simulink model "quadcopter_model"  (R2023a)
settings: Solver=odeN  StartTime=0.0  StopTime=20  MaxStep=0.2  RelTol=1e-3
libraries: slpidlib x3
settings Model: Creator=Lenovo  LastModifiedBy=Lenovo
settings SolverCC: MaxConsecutiveMinStep=5

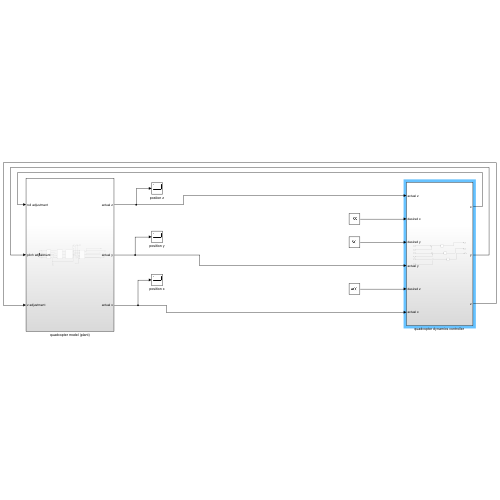
[thumbnail: Simulink's stored preview of the top-level diagram]
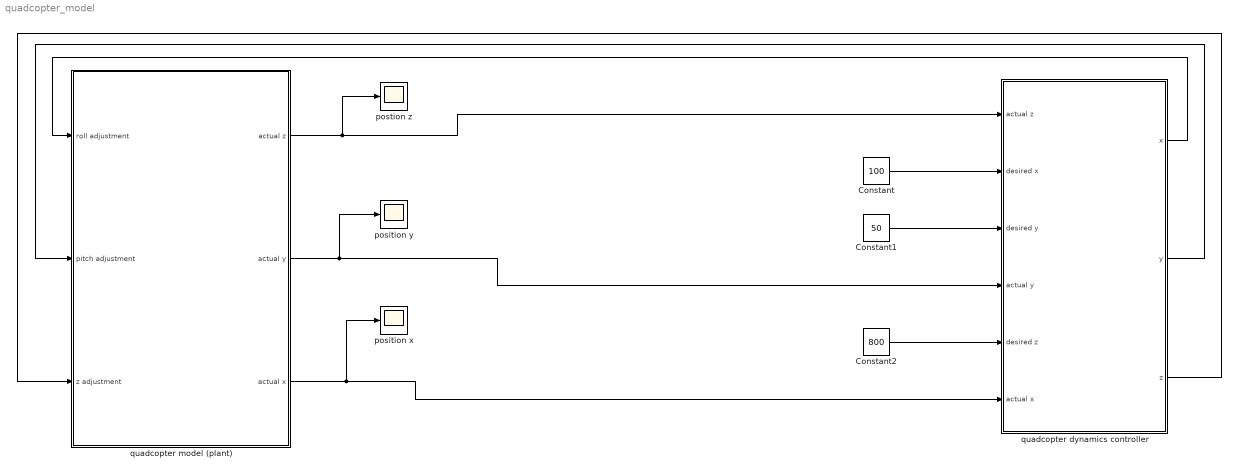
== system quadcopter_model ==
  Constant : Constant  Value=100
  Constant1 : Constant  Value=50
  Constant2 : Constant  Value=800
  position x : Scope
  position y : Scope
  postion z : Scope
  "quadcopter dynamics controller " : Subsystem
  quadcopter model (plant) : Subsystem
  wires:
  "quadcopter dynamics controller "/3(z) -> quadcopter model (plant)/3(z adjustment)
  "quadcopter dynamics controller "/2(y) -> quadcopter model (plant)/2("pitch adjustment ")
  "quadcopter dynamics controller "/1(x) -> quadcopter model (plant)/1(roll adjustment)
  quadcopter model (plant)/1(actual z) -> postion z/1, "quadcopter dynamics controller "/1(actual z)
  quadcopter model (plant)/2(actual y) -> position y/1, "quadcopter dynamics controller "/4(actual y)
  quadcopter model (plant)/3(actual x) -> position x/1, "quadcopter dynamics controller "/6(actual x)
  Constant1/1 -> "quadcopter dynamics controller "/3(desired y)
  Constant/1 -> "quadcopter dynamics controller "/2(desired x)
  Constant2/1 -> "quadcopter dynamics controller "/5(desired z)

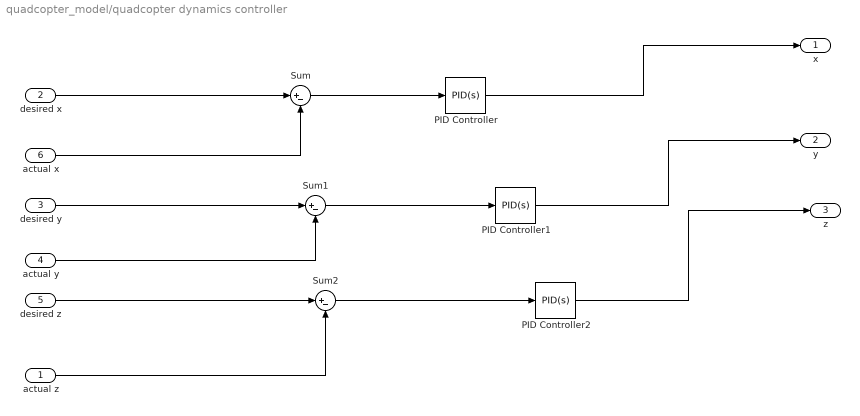
== system quadcopter_model/quadcopter dynamics controller  ==
  actual z : Inport
  desired x : Inport  Port=2
  desired y : Inport  Port=3
  actual y : Inport  Port=4
  desired z : Inport  Port=5
  actual x : Inport  Port=6
  PID Controller : slpidlib/PID Controller  Controller=PID  Form=Parallel  TimeDomain=Continuous-time  UseExternalTs=off  SampleTime=-1  IntegratorMethod=Forward Euler  FilterMethod=Forward Euler  ControllerParametersSource=internal  P=5.80247697722311e-07  I=2.71641673162191e-08  UseKiTs=on  D=3.04350306749436e-06  N=5.45397025421619  UseFilter=on  TunerSelectOption=Transfer Function Based (PID Tuner App)  InitialConditionSource=internal  InitialConditionForIntegrator=0  InitialConditionForFilter=0  DifferentiatorICPrevScaledInput=0  ExternalReset=none  TrackingMode=off  Kt=1  LimitOutput=off  SatLimitsSource=internal  UpperSaturationLimit=inf  LowerSaturationLimit=-inf  LinearizeAsGain=on  AntiWindupMode=none  Kb=1  LimitIntegrator=off  UpperIntegratorSaturationLimit=inf  LowerIntegratorSaturationLimit=-inf  POutMin=[]  POutMax=[]  IOutMin=[]  IOutMax=[]  DOutMin=[]  DOutMax=[]  NOutMin=[]  NOutMax=[]  SumOutMin=[]  SumOutMax=[]  SaturationOutMin=[]  SaturationOutMax=[]  PParamMin=[]  PParamMax=[]  IParamMin=[]  IParamMax=[]  DParamMin=[]  DParamMax=[]  NParamMin=[]  NParamMax=[]  KbParamMin=[]  KbParamMax=[]  KtParamMin=[]  KtParamMax=[]  KbOutMin=[]  KbOutMax=[]  KtOutMin=[]  KtOutMax=[]  IntegratorOutMin=[]  IntegratorOutMax=[]  FilterOutMin=[]  FilterOutMax=[]  SumI1OutMin=[]  SumI1OutMax=[]  SumI2OutMin=[]  SumI2OutMax=[]  SumI3OutMin=[]  SumI3OutMax=[]  SumI4OutMin=[]  SumI4OutMax=[]  SumDOutMin=[]  SumDOutMax=[]  DifferentiatorOutMin=[]  DifferentiatorOutMax=[]  FilterDiffOutCoefMin=[]  FilterDiffOutCoefMax=[]  ReciprocalOutMin=[]  ReciprocalOutMax=[]  SumDenOutMin=[]  SumDenOutMax=[]  SumNumOutMin=[]  SumNumOutMax=[]  DivideOutMin=[]  DivideOutMax=[]  UdiffTsProdOutMin=[]  UdiffTsProdOutMax=[]  NTsProdOutMin=[]  NTsProdOutMax=[]  UintegralTsProdOutMin=[]  UintegralTsProdOutMax=[]  UngainTsProdOutMin=[]  UngainTsProdOutMax=[]  ClampingZeroOutDataTypeStr=Inherit: Inherit via back propagation  ClampingZeroOutMin=[]  ClampingZeroOutMax=[]  FilterDenConstantOutDataTypeStr=Inherit: Inherit via back propagation  FilterDenConstantOutMin=[]  FilterDenConstantOutMax=[]  PCopyOutDataTypeStr=Inherit: Inherit via back propagation  PCopyOutMin=[]  PCopyOutMax=[]  NCopyOutDataTypeStr=Inherit: Inherit via back propagation  NCopyOutMin=[]  NCopyOutMax=[]  IntegratorContinuousStateAttributes=''  IntegratorStateMustResolveToSignalObject=off  IntegratorRTWStateStorageClass=Auto  FilterContinuousStateAttributes=''  FilterStateMustResolveToSignalObject=off  FilterRTWStateStorageClass=Auto  ParallelPVariant=InternalParameters  IdealPVariant=Disabled  IVariant=InternalParameters  DVariant=InternalParameters  IntegratorVariant=Continuous  SatVariant=Disabled  AWVariant=Passthrough  PCopyVariant=Disabled  TRVariant=Disabled  FdbkBlocksVariant=Forward  IdealPFdbkVariant=Disabled  SatFdbkVariant=Disabled  DerivativeFilterVariant=ContFilter  NVariant=InternalParameters  NCopyVariant=Disabled  FilterICVariant=InternalICsFilter  IntegratorICVariant=InternalICs  ExternalResetVariant=Disabled  TRSumVariant=Passthrough  SumFdbkVariant=Disabled  SumVariant=Sum_PID  TsampFilterVariant=InternalTs  TsampNgainVariant=Passthrough  TsampIntegralVariant=Disabled_SignalSpec  ExternalSaturationOutDataTypeStr=Inherit: Same as second input
  PID Controller1 : slpidlib/PID Controller  Controller=PID  Form=Ideal  TimeDomain=Continuous-time  UseExternalTs=off  SampleTime=-1  IntegratorMethod=Forward Euler  FilterMethod=Forward Euler  ControllerParametersSource=internal  P=-5.80247697722311e-07  I=0.0468147782797737  UseKiTs=on  D=5.24517904929436  N=5.45397025421619  UseFilter=on  TunerSelectOption=Transfer Function Based (PID Tuner App)  InitialConditionSource=internal  InitialConditionForIntegrator=0  InitialConditionForFilter=0  DifferentiatorICPrevScaledInput=0  ExternalReset=none  TrackingMode=off  Kt=1  LimitOutput=off  SatLimitsSource=internal  UpperSaturationLimit=inf  LowerSaturationLimit=-inf  LinearizeAsGain=on  AntiWindupMode=none  Kb=1  LimitIntegrator=off  UpperIntegratorSaturationLimit=inf  LowerIntegratorSaturationLimit=-inf  POutMin=[]  POutMax=[]  IOutMin=[]  IOutMax=[]  DOutMin=[]  DOutMax=[]  NOutMin=[]  NOutMax=[]  SumOutMin=[]  SumOutMax=[]  SaturationOutMin=[]  SaturationOutMax=[]  PParamMin=[]  PParamMax=[]  IParamMin=[]  IParamMax=[]  DParamMin=[]  DParamMax=[]  NParamMin=[]  NParamMax=[]  KbParamMin=[]  KbParamMax=[]  KtParamMin=[]  KtParamMax=[]  KbOutMin=[]  KbOutMax=[]  KtOutMin=[]  KtOutMax=[]  IntegratorOutMin=[]  IntegratorOutMax=[]  FilterOutMin=[]  FilterOutMax=[]  SumI1OutMin=[]  SumI1OutMax=[]  SumI2OutMin=[]  SumI2OutMax=[]  SumI3OutMin=[]  SumI3OutMax=[]  SumI4OutMin=[]  SumI4OutMax=[]  SumDOutMin=[]  SumDOutMax=[]  DifferentiatorOutMin=[]  DifferentiatorOutMax=[]  FilterDiffOutCoefMin=[]  FilterDiffOutCoefMax=[]  ReciprocalOutMin=[]  ReciprocalOutMax=[]  SumDenOutMin=[]  SumDenOutMax=[]  SumNumOutMin=[]  SumNumOutMax=[]  DivideOutMin=[]  DivideOutMax=[]  UdiffTsProdOutMin=[]  UdiffTsProdOutMax=[]  NTsProdOutMin=[]  NTsProdOutMax=[]  UintegralTsProdOutMin=[]  UintegralTsProdOutMax=[]  UngainTsProdOutMin=[]  UngainTsProdOutMax=[]  ClampingZeroOutDataTypeStr=Inherit: Inherit via back propagation  ClampingZeroOutMin=[]  ClampingZeroOutMax=[]  FilterDenConstantOutDataTypeStr=Inherit: Inherit via back propagation  FilterDenConstantOutMin=[]  FilterDenConstantOutMax=[]  PCopyOutDataTypeStr=Inherit: Inherit via back propagation  PCopyOutMin=[]  PCopyOutMax=[]  NCopyOutDataTypeStr=Inherit: Inherit via back propagation  NCopyOutMin=[]  NCopyOutMax=[]  IntegratorContinuousStateAttributes=''  IntegratorStateMustResolveToSignalObject=off  IntegratorRTWStateStorageClass=Auto  FilterContinuousStateAttributes=''  FilterStateMustResolveToSignalObject=off  FilterRTWStateStorageClass=Auto  ParallelPVariant=Passthrough  IdealPVariant=InternalParameters  IVariant=InternalParameters  DVariant=InternalParameters  IntegratorVariant=Continuous  SatVariant=Disabled  AWVariant=Passthrough  PCopyVariant=Disabled  TRVariant=Disabled  FdbkBlocksVariant=Forward  IdealPFdbkVariant=Disabled  SatFdbkVariant=Disabled  DerivativeFilterVariant=ContFilter  NVariant=InternalParameters  NCopyVariant=Disabled  FilterICVariant=InternalICsFilter  IntegratorICVariant=InternalICs  ExternalResetVariant=Disabled  TRSumVariant=Passthrough  SumFdbkVariant=Disabled  SumVariant=Sum_PID  TsampFilterVariant=InternalTs  TsampNgainVariant=Passthrough  TsampIntegralVariant=Disabled_SignalSpec  ExternalSaturationOutDataTypeStr=Inherit: Same as second input
  PID Controller2 : slpidlib/PID Controller  Controller=PID  Form=Parallel  TimeDomain=Continuous-time  UseExternalTs=off  SampleTime=-1  IntegratorMethod=Forward Euler  FilterMethod=Forward Euler  ControllerParametersSource=internal  P=5.80247697722311e-07  I=2.71641673162191e-08  UseKiTs=off  D=3.04350306749436e-06  N=5.45397025421619  UseFilter=on  TunerSelectOption=Transfer Function Based (PID Tuner App)  InitialConditionSource=internal  InitialConditionForIntegrator=0  InitialConditionForFilter=0  DifferentiatorICPrevScaledInput=0  ExternalReset=none  TrackingMode=off  Kt=1  LimitOutput=off  SatLimitsSource=internal  UpperSaturationLimit=inf  LowerSaturationLimit=-inf  LinearizeAsGain=on  AntiWindupMode=none  Kb=1  LimitIntegrator=off  UpperIntegratorSaturationLimit=inf  LowerIntegratorSaturationLimit=-inf  POutMin=[]  POutMax=[]  IOutMin=[]  IOutMax=[]  DOutMin=[]  DOutMax=[]  NOutMin=[]  NOutMax=[]  SumOutMin=[]  SumOutMax=[]  SaturationOutMin=[]  SaturationOutMax=[]  PParamMin=[]  PParamMax=[]  IParamMin=[]  IParamMax=[]  DParamMin=[]  DParamMax=[]  NParamMin=[]  NParamMax=[]  KbParamMin=[]  KbParamMax=[]  KtParamMin=[]  KtParamMax=[]  KbOutMin=[]  KbOutMax=[]  KtOutMin=[]  KtOutMax=[]  IntegratorOutMin=[]  IntegratorOutMax=[]  FilterOutMin=[]  FilterOutMax=[]  SumI1OutMin=[]  SumI1OutMax=[]  SumI2OutMin=[]  SumI2OutMax=[]  SumI3OutMin=[]  SumI3OutMax=[]  SumI4OutMin=[]  SumI4OutMax=[]  SumDOutMin=[]  SumDOutMax=[]  DifferentiatorOutMin=[]  DifferentiatorOutMax=[]  FilterDiffOutCoefMin=[]  FilterDiffOutCoefMax=[]  ReciprocalOutMin=[]  ReciprocalOutMax=[]  SumDenOutMin=[]  SumDenOutMax=[]  SumNumOutMin=[]  SumNumOutMax=[]  DivideOutMin=[]  DivideOutMax=[]  UdiffTsProdOutMin=[]  UdiffTsProdOutMax=[]  NTsProdOutMin=[]  NTsProdOutMax=[]  UintegralTsProdOutMin=[]  UintegralTsProdOutMax=[]  UngainTsProdOutMin=[]  UngainTsProdOutMax=[]  ClampingZeroOutDataTypeStr=Inherit: Inherit via back propagation  ClampingZeroOutMin=[]  ClampingZeroOutMax=[]  FilterDenConstantOutDataTypeStr=Inherit: Inherit via back propagation  FilterDenConstantOutMin=[]  FilterDenConstantOutMax=[]  PCopyOutDataTypeStr=Inherit: Inherit via back propagation  PCopyOutMin=[]  PCopyOutMax=[]  NCopyOutDataTypeStr=Inherit: Inherit via back propagation  NCopyOutMin=[]  NCopyOutMax=[]  IntegratorContinuousStateAttributes=''  IntegratorStateMustResolveToSignalObject=off  IntegratorRTWStateStorageClass=Auto  FilterContinuousStateAttributes=''  FilterStateMustResolveToSignalObject=off  FilterRTWStateStorageClass=Auto  ParallelPVariant=InternalParameters  IdealPVariant=Disabled  IVariant=InternalParameters  DVariant=InternalParameters  IntegratorVariant=Continuous  SatVariant=Disabled  AWVariant=Passthrough  PCopyVariant=Disabled  TRVariant=Disabled  FdbkBlocksVariant=Forward  IdealPFdbkVariant=Disabled  SatFdbkVariant=Disabled  DerivativeFilterVariant=ContFilter  NVariant=InternalParameters  NCopyVariant=Disabled  FilterICVariant=InternalICsFilter  IntegratorICVariant=InternalICs  ExternalResetVariant=Disabled  TRSumVariant=Passthrough  SumFdbkVariant=Disabled  SumVariant=Sum_PID  TsampFilterVariant=InternalTs  TsampNgainVariant=Passthrough  TsampIntegralVariant=Disabled_SignalSpec  ExternalSaturationOutDataTypeStr=Inherit: Same as second input
  Sum : Sum  Inputs=|+-
  Sum1 : Sum  Inputs=|+-
  Sum2 : Sum  Inputs=|+-
  x : Outport
  y : Outport  Port=2
  z : Outport  Port=3
  wires:
  desired x/1 -> Sum/1
  actual x/1 -> Sum/2
  desired y/1 -> Sum1/1
  actual y/1 -> Sum1/2
  actual z/1 -> Sum2/2
  desired z/1 -> Sum2/1
  Sum1/1 -> PID Controller1/1
  Sum/1 -> PID Controller/1
  Sum2/1 -> PID Controller2/1
  PID Controller2/1 -> z/1
  PID Controller1/1 -> y/1
  PID Controller/1 -> x/1

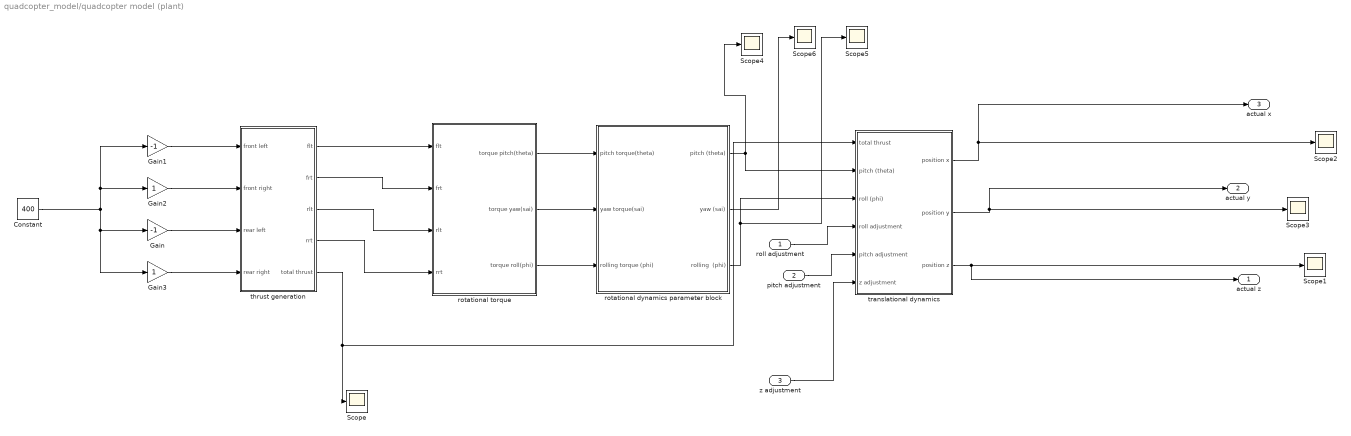
== system quadcopter_model/quadcopter model (plant) ==
  roll adjustment : Inport
  "pitch adjustment " : Inport  Port=2
  z adjustment : Inport  Port=3
  Constant : Constant  Value=400
  Gain : Gain  Gain=-1
  Gain1 : Gain  Gain=-1
  Gain2 : Gain
  Gain3 : Gain
  Scope{,1..6} (7 alike) : Scope
  rotational dynamics parameter block : Subsystem
  rotational torque : Subsystem
  thrust generation : Subsystem
  translational dynamics : Subsystem
  actual z : Outport
  actual y : Outport  Port=2
  actual x : Outport  Port=3
  wires:
  Gain3/1 -> thrust generation/4(rear right)
  translational dynamics/3(position z) -> Scope1/1, actual z/1
  translational dynamics/1(position x) -> Scope2/1, actual x/1
  translational dynamics/2(position y) -> actual y/1, Scope3/1
  rotational dynamics parameter block/2(yaw (sai)) -> Scope6/1
  Gain/1 -> thrust generation/3(rear left)
  rotational dynamics parameter block/1(pitch (theta)) -> translational dynamics/2("pitch (theta) "), Scope4/1
  rotational torque/1(torque pitch(theta)) -> rotational dynamics parameter block/1(pitch torque(theta))
  rotational torque/2(torque yaw(sai)) -> rotational dynamics parameter block/2(yaw torque(sai))
  Gain2/1 -> thrust generation/2(front right)
  thrust generation/3(rlt) -> rotational torque/3(rlt)
  thrust generation/4(rrt) -> rotational torque/4(rrt)
  thrust generation/1(flt) -> rotational torque/1(flt)
  Gain1/1 -> thrust generation/1(front left)
  rotational torque/3(torque roll(phi)) -> rotational dynamics parameter block/3(rolling torque (phi))
  thrust generation/2(frt) -> rotational torque/2(frt)
  Constant/1 -> Gain3/1, Gain/1, Gain2/1, Gain1/1
  thrust generation/5("total thrust ") -> translational dynamics/1(total thrust), Scope/1
  z adjustment/1 -> translational dynamics/6(z adjustment)
  roll adjustment/1 -> translational dynamics/4(roll adjustment)
  "pitch adjustment "/1 -> translational dynamics/5(pitch adjustment)
  rotational dynamics parameter block/3(rolling  (phi)) -> Scope5/1, translational dynamics/3(roll (phi))

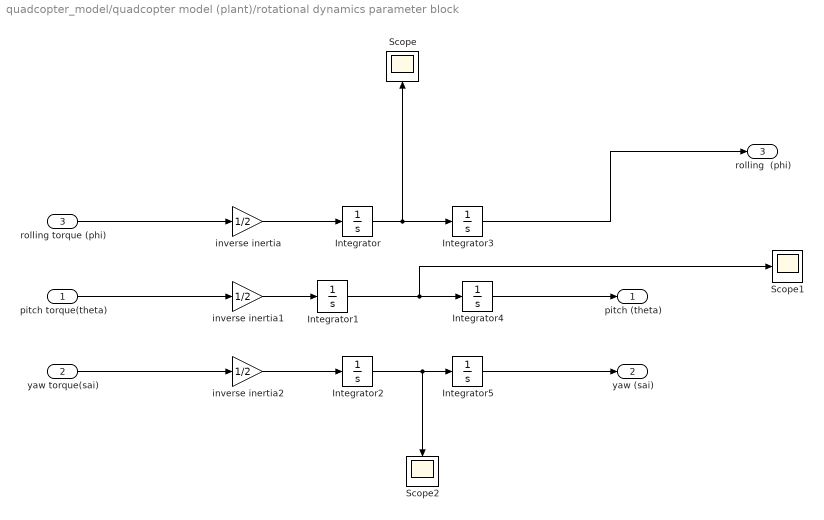
== system quadcopter_model/quadcopter model (plant)/rotational dynamics parameter block ==
  pitch torque(theta) : Inport
  yaw torque(sai) : Inport  Port=2
  rolling torque (phi) : Inport  Port=3
  Integrator{,2..5} (5 alike) : Integrator
  Integrator1 : Integrator  LimitOutput=on  UpperSaturationLimit=750  LowerSaturationLimit=-750  IgnoreLimit=on
  Scope : Scope
  Scope1 : Scope
  Scope2 : Scope
  inverse inertia : Gain  Gain=1/2
  inverse inertia1 : Gain  Gain=1/2
  inverse inertia2 : Gain  Gain=1/2
  pitch (theta) : Outport
  yaw (sai) : Outport  Port=2
  rolling  (phi) : Outport  Port=3
  wires:
  rolling torque (phi)/1 -> inverse inertia/1
  pitch torque(theta)/1 -> inverse inertia1/1
  yaw torque(sai)/1 -> inverse inertia2/1
  inverse inertia1/1 -> Integrator1/1
  inverse inertia2/1 -> Integrator2/1
  inverse inertia/1 -> Integrator/1
  Integrator/1 -> Scope/1, Integrator3/1
  Integrator2/1 -> Scope2/1, Integrator5/1
  Integrator5/1 -> yaw (sai)/1
  Integrator1/1 -> Scope1/1, Integrator4/1
  Integrator3/1 -> rolling  (phi)/1
  Integrator4/1 -> pitch (theta)/1

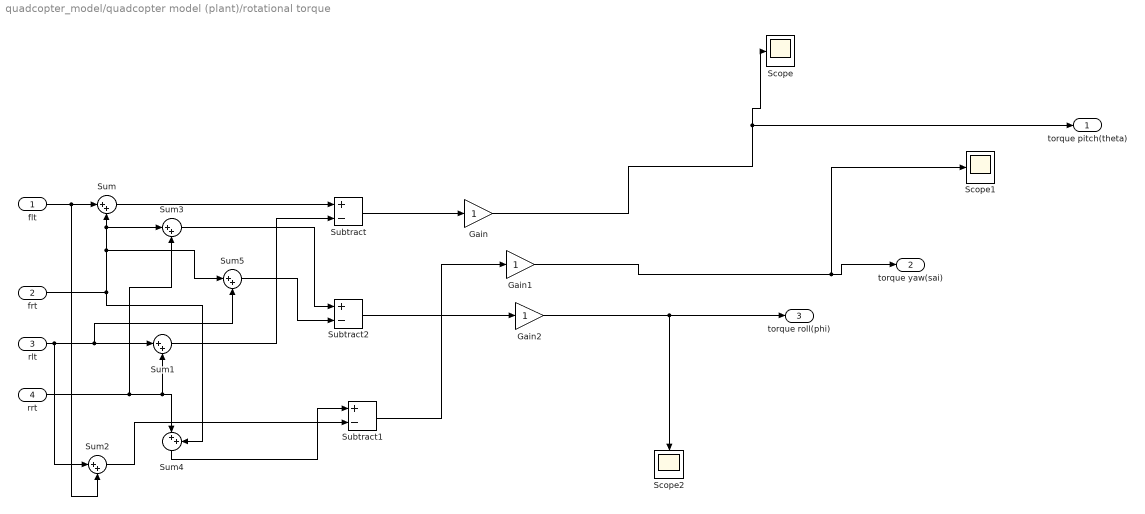
== system quadcopter_model/quadcopter model (plant)/rotational torque ==
  flt : Inport
  frt : Inport  Port=2
  rlt : Inport  Port=3
  rrt : Inport  Port=4
  Gain : Gain
  Gain1 : Gain
  Gain2 : Gain
  Scope : Scope
  Scope1 : Scope
  Scope2 : Scope
  Subtract : Sum  Inputs=+-
  Subtract1 : Sum  Inputs=+-
  Subtract2 : Sum  Inputs=+-
  Sum{,1..5} (6 alike) : Sum  Inputs=|++
  torque pitch(theta) : Outport
  torque yaw(sai) : Outport  Port=2
  torque roll(phi) : Outport  Port=3
  wires:
  frt/1 -> Sum4/2, Sum3/1, Sum/2, Sum5/1
  flt/1 -> Sum/1, Sum2/2
  rlt/1 -> Sum1/1, Sum5/2, Sum2/1
  rrt/1 -> Sum3/2, Sum4/1, Sum1/2
  Sum/1 -> Subtract/1
  Sum1/1 -> Subtract/2
  Subtract/1 -> Gain/1
  Subtract1/1 -> Gain1/1
  Sum3/1 -> Subtract2/1
  Sum5/1 -> Subtract2/2
  Subtract2/1 -> Gain2/1
  Sum2/1 -> Subtract1/2
  Sum4/1 -> Subtract1/1
  Gain1/1 -> Scope1/1, torque yaw(sai)/1
  Gain/1 -> torque pitch(theta)/1, Scope/1
  Gain2/1 -> torque roll(phi)/1, Scope2/1

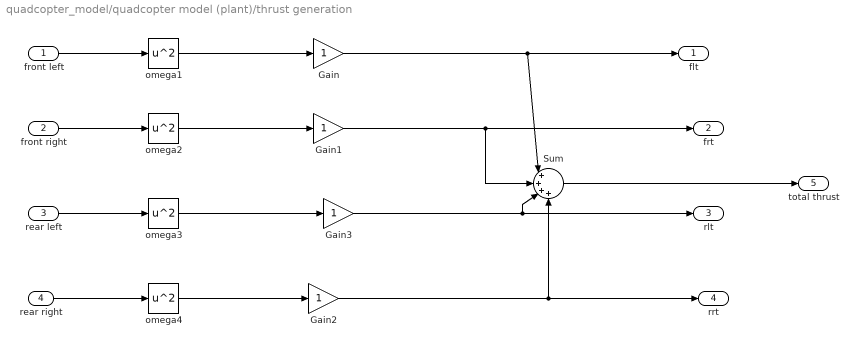
== system quadcopter_model/quadcopter model (plant)/thrust generation ==
  front left : Inport
  front right : Inport  Port=2
  rear left : Inport  Port=3
  rear right : Inport  Port=4
  Gain{,1..3} (4 alike) : Gain
  Sum : Sum  Inputs=|++++
  omega1 : Math  Operator=square  OutputSignalType=real
  omega2 : Math  Operator=square
  omega3 : Math  Operator=square
  omega4 : Math  Operator=square
  flt : Outport
  frt : Outport  Port=2
  rlt : Outport  Port=3
  rrt : Outport  Port=4
  "total thrust " : Outport  Port=5
  wires:
  front left/1 -> omega1/1
  front right/1 -> omega2/1
  rear left/1 -> omega3/1
  rear right/1 -> omega4/1
  omega1/1 -> Gain/1
  omega3/1 -> Gain3/1
  Sum/1 -> "total thrust "/1
  omega4/1 -> Gain2/1
  omega2/1 -> Gain1/1
  Gain/1 -> Sum/1, flt/1
  Gain1/1 -> Sum/2, frt/1
  Gain2/1 -> Sum/4, rrt/1
  Gain3/1 -> Sum/3, rlt/1

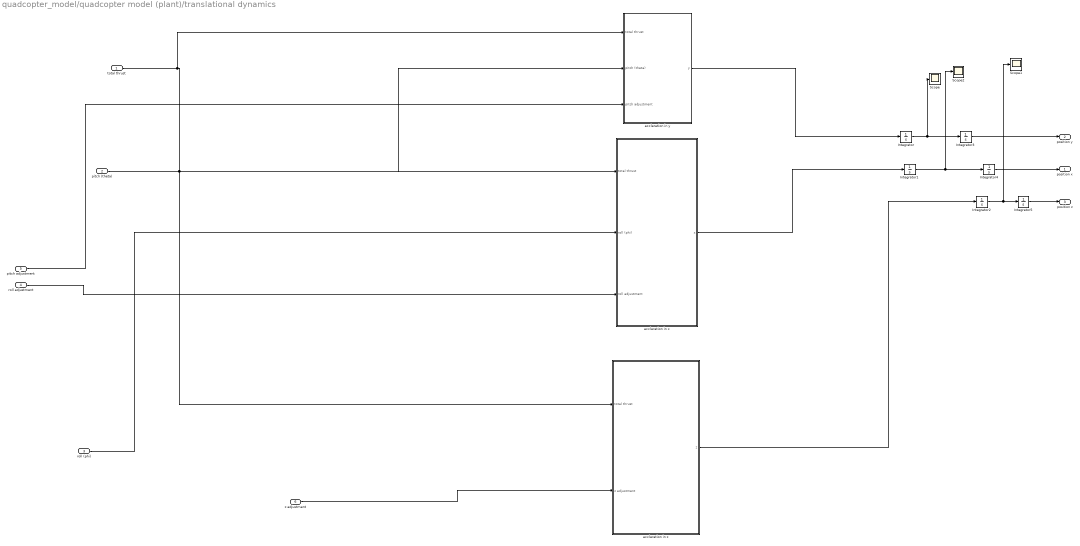
== system quadcopter_model/quadcopter model (plant)/translational dynamics ==
  total thrust : Inport
  "pitch (theta) " : Inport  Port=2
  roll (phi) : Inport  Port=3
  roll adjustment : Inport  Port=4
  pitch adjustment : Inport  Port=5
  z adjustment : Inport  Port=6
  Integrator{,1..5} (6 alike) : Integrator
  Scope : Scope
  Scope1 : Scope
  Scope2 : Scope
  accleration in x : Subsystem
  accleration in y : Subsystem
  accleration in z : Subsystem
  position x : Outport
  position y : Outport  Port=2
  position z : Outport  Port=3
  wires:
  total thrust/1 -> accleration in y/1(total thrust), accleration in z/1(total thrust), accleration in x/1(total thrust)
  "pitch (theta) "/1 -> accleration in y/2("pitch (theta) ")
  roll (phi)/1 -> accleration in x/2(roll (phi))
  accleration in y/1(y) -> Integrator/1
  accleration in x/1(x) -> Integrator1/1
  accleration in z/1(z) -> Integrator2/1
  Integrator/1 -> Scope/1, Integrator3/1
  Integrator1/1 -> Scope2/1, Integrator4/1
  Integrator2/1 -> Scope1/1, Integrator5/1
  Integrator3/1 -> position y/1
  Integrator4/1 -> position x/1
  Integrator5/1 -> position z/1
  pitch adjustment/1 -> accleration in y/3(pitch adjustment)
  roll adjustment/1 -> accleration in x/3(roll adjustment)
  z adjustment/1 -> accleration in z/2(z adjustment)

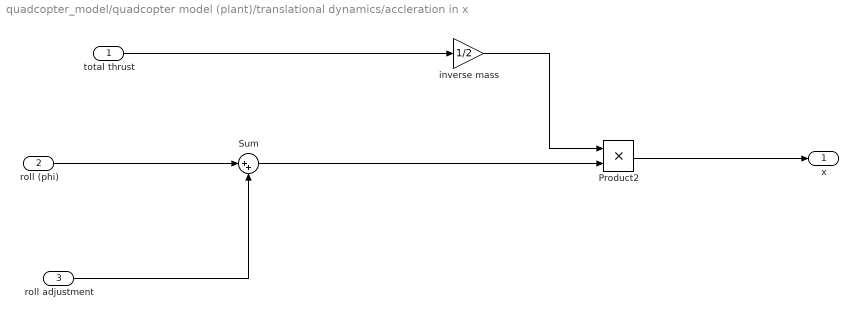
== system quadcopter_model/quadcopter model (plant)/translational dynamics/accleration in x ==
  total thrust : Inport
  roll (phi) : Inport  Port=2
  roll adjustment : Inport  Port=3
  Product2 : Product
  Sum : Sum  Inputs=|++
  inverse mass : Gain  Gain=1/2
  x : Outport
  wires:
  total thrust/1 -> inverse mass/1
  inverse mass/1 -> Product2/1
  Product2/1 -> x/1
  roll adjustment/1 -> Sum/2
  roll (phi)/1 -> Sum/1
  Sum/1 -> Product2/2

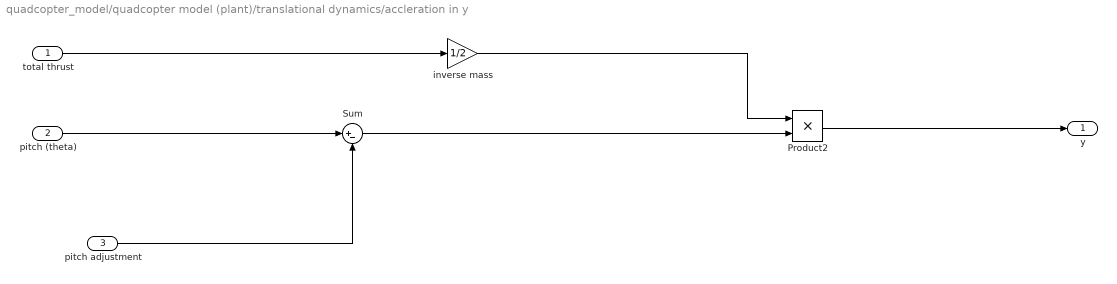
== system quadcopter_model/quadcopter model (plant)/translational dynamics/accleration in y ==
  total thrust : Inport
  "pitch (theta) " : Inport  Port=2
  pitch adjustment : Inport  Port=3
  Product2 : Product
  Sum : Sum  Inputs=|+-
  inverse mass : Gain  Gain=1/2
  y : Outport
  wires:
  Product2/1 -> y/1
  total thrust/1 -> inverse mass/1
  inverse mass/1 -> Product2/1
  pitch adjustment/1 -> Sum/2
  "pitch (theta) "/1 -> Sum/1
  Sum/1 -> Product2/2

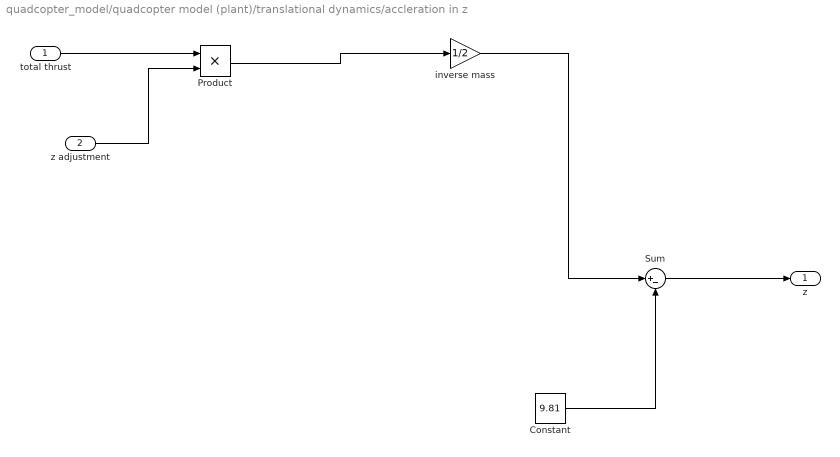
== system quadcopter_model/quadcopter model (plant)/translational dynamics/accleration in z ==
  total thrust : Inport
  z adjustment : Inport  Port=2
  Constant : Constant  Value=9.81
  Product : Product
  Sum : Sum  Inputs=|+-
  inverse mass : Gain  Gain=1/2
  z : Outport
  wires:
  Constant/1 -> Sum/2
  Sum/1 -> z/1
  inverse mass/1 -> Sum/1
  total thrust/1 -> Product/1
  z adjustment/1 -> Product/2
  Product/1 -> inverse mass/1
